simulink model "sliding_mode_controller_2014b"  (R2021b)
settings: Solver=ode3  StartTime=0.0  StopTime=30  FixedStep=0.01  RelTol=1e-3  EnableMultiTasking=on
model workspace (MAT data in the model file):
  P_C_1 = Simulink.Signal
  P_C_1.DataType = 'double'
  P_C_1.Dimensions = 1
  P_C_1.DimensionsMode = 'Fixed'
  P_C_1.Complexity = 'real'
  P_C_1.SampleTime = -1
  P_C_1.SamplingMode = 'Sample based'
  P_C_1.InitialValue = '0'
  P_C_2 = Simulink.Signal
  P_C_2.DataType = 'double'
  P_C_2.Dimensions = 1
  P_C_2.DimensionsMode = 'Fixed'
  P_C_2.Complexity = 'real'
  P_C_2.SampleTime = -1
  P_C_2.SamplingMode = 'Sample based'
  P_C_2.InitialValue = '0'
  P_C_3 = Simulink.Signal
  P_C_3.DataType = 'double'
  P_C_3.Dimensions = 1
  P_C_3.DimensionsMode = 'Fixed'
  P_C_3.Complexity = 'real'
  P_C_3.SampleTime = -1
  P_C_3.SamplingMode = 'Sample based'
  P_C_3.InitialValue = '0'
  P_C_4 = Simulink.Signal
  P_C_4.DataType = 'double'
  P_C_4.Dimensions = 1
  P_C_4.DimensionsMode = 'Fixed'
  P_C_4.Complexity = 'real'
  P_C_4.SampleTime = -1
  P_C_4.SamplingMode = 'Sample based'
  P_C_4.InitialValue = '0'
  alfa_1 = Simulink.Signal
  alfa_1.DataType = 'double'
  alfa_1.Dimensions = 1
  alfa_1.DimensionsMode = 'Fixed'
  alfa_1.Complexity = 'real'
  alfa_1.SampleTime = -1
  alfa_1.SamplingMode = 'Sample based'
  alfa_1.InitialValue = '0'
  alfa_2 = Simulink.Signal
  alfa_2.DataType = 'double'
  alfa_2.Dimensions = 1
  alfa_2.DimensionsMode = 'Fixed'
  alfa_2.Complexity = 'real'
  alfa_2.SampleTime = -1
  alfa_2.SamplingMode = 'Sample based'
  alfa_2.InitialValue = '0'
  alfa_3 = Simulink.Signal
  alfa_3.DataType = 'double'
  alfa_3.Dimensions = 1
  alfa_3.DimensionsMode = 'Fixed'
  alfa_3.Complexity = 'real'
  alfa_3.SampleTime = -1
  alfa_3.SamplingMode = 'Sample based'
  alfa_3.InitialValue = '0'
  counter_1 = Simulink.Signal
  counter_1.DataType = 'double'
  counter_1.Dimensions = 1
  counter_1.DimensionsMode = 'Fixed'
  counter_1.Complexity = 'real'
  counter_1.SampleTime = -1
  counter_1.SamplingMode = 'Sample based'
  counter_1.InitialValue = '0'
  counter_2 = Simulink.Signal
  counter_2.DataType = 'double'
  counter_2.Dimensions = 1
  counter_2.DimensionsMode = 'Fixed'
  counter_2.Complexity = 'real'
  counter_2.SampleTime = -1
  counter_2.SamplingMode = 'Sample based'
  counter_2.InitialValue = '0'
  counter_3 = Simulink.Signal
  counter_3.DataType = 'double'
  counter_3.Dimensions = 1
  counter_3.DimensionsMode = 'Fixed'
  counter_3.Complexity = 'real'
  counter_3.SampleTime = -1
  counter_3.SamplingMode = 'Sample based'
  counter_3.InitialValue = '0'
  counter_4 = Simulink.Signal
  counter_4.DataType = 'double'
  counter_4.Dimensions = 1
  counter_4.DimensionsMode = 'Fixed'
  counter_4.Complexity = 'real'
  counter_4.SampleTime = -1
  counter_4.SamplingMode = 'Sample based'
  counter_4.InitialValue = '0'
  lambda_1 = Simulink.Signal
  lambda_1.DataType = 'double'
  lambda_1.Dimensions = 1
  lambda_1.DimensionsMode = 'Fixed'
  lambda_1.Complexity = 'real'
  lambda_1.SampleTime = -1
  lambda_1.SamplingMode = 'Sample based'
  lambda_1.InitialValue = '0'
  lambda_2 = Simulink.Signal
  lambda_2.DataType = 'double'
  lambda_2.Dimensions = 1
  lambda_2.DimensionsMode = 'Fixed'
  lambda_2.Complexity = 'real'
  lambda_2.SampleTime = -1
  lambda_2.SamplingMode = 'Sample based'
  lambda_2.InitialValue = '0'
  lambda_3 = Simulink.Signal
  lambda_3.DataType = 'double'
  lambda_3.Dimensions = 1
  lambda_3.DimensionsMode = 'Fixed'
  lambda_3.Complexity = 'real'
  lambda_3.SampleTime = -1
  lambda_3.SamplingMode = 'Sample based'
  lambda_3.InitialValue = '0'
  mf_1 = Simulink.Signal
  mf_1.DataType = 'double'
  mf_1.Dimensions = 1
  mf_1.DimensionsMode = 'Fixed'
  mf_1.Complexity = 'real'
  mf_1.SampleTime = -1
  mf_1.SamplingMode = 'Sample based'
  mf_1.InitialValue = '.5'
  mf_2 = Simulink.Signal
  mf_2.DataType = 'double'
  mf_2.Dimensions = 1
  mf_2.DimensionsMode = 'Fixed'
  mf_2.Complexity = 'real'
  mf_2.SampleTime = -1
  mf_2.SamplingMode = 'Sample based'
  mf_2.InitialValue = '.5'
  mf_3 = Simulink.Signal
  mf_3.DataType = 'double'
  mf_3.Dimensions = 1
  mf_3.DimensionsMode = 'Fixed'
  mf_3.Complexity = 'real'
  mf_3.SampleTime = -1
  mf_3.SamplingMode = 'Sample based'
  mf_3.InitialValue = '.5'
  step_counter = Simulink.Signal
  step_counter.DataType = 'double'
  step_counter.Dimensions = 1
  step_counter.DimensionsMode = 'auto'
  step_counter.Complexity = 'real'
  step_counter.SampleTime = -1
  step_counter.SamplingMode = 'auto'
  step_counter.InitialValue = '0'
  trans_b_1 = Simulink.Signal
  trans_b_1.DataType = 'double'
  trans_b_1.Dimensions = 1
  trans_b_1.DimensionsMode = 'Fixed'
  trans_b_1.Complexity = 'real'
  trans_b_1.SampleTime = -1
  trans_b_1.SamplingMode = 'Sample based'
  trans_b_1.InitialValue = '0'
  trans_b_2 = Simulink.Signal
  trans_b_2.DataType = 'double'
  trans_b_2.Dimensions = 1
  trans_b_2.DimensionsMode = 'Fixed'
  trans_b_2.Complexity = 'real'
  trans_b_2.SampleTime = -1
  trans_b_2.SamplingMode = 'Sample based'
  trans_b_2.InitialValue = '0'
  trans_b_3 = Simulink.Signal
  trans_b_3.DataType = 'double'
  trans_b_3.Dimensions = 1
  trans_b_3.DimensionsMode = 'Fixed'
  trans_b_3.Complexity = 'real'
  trans_b_3.SampleTime = -1
  trans_b_3.SamplingMode = 'Sample based'
  trans_b_3.InitialValue = '0'
  trans_b_4 = Simulink.Signal
  trans_b_4.DataType = 'double'
  trans_b_4.Dimensions = 1
  trans_b_4.DimensionsMode = 'Fixed'
  trans_b_4.Complexity = 'real'
  trans_b_4.SampleTime = -1
  trans_b_4.SamplingMode = 'Sample based'
  trans_b_4.InitialValue = '0'
values from neighbouring files (symbols this model uses):
  alfa0 = 15*pi/180    (= 0.261799387799)    [engine_initials_smc.m]
  etaif2 = -0.015    [engine_initials_smc.m]
  Hu = 43000    [engine_initials_smc.m]
  I = Iac*(2.0*pi/60)^2*1000    (= 5.26378901391)    [engine_initials_smc.m]
  kb2 = 0.470    (= 0.47)    [engine_initials_smc.m]
  Lth = 14.67    [engine_initials_smc.m]
  mat1 = 5.9403    [engine_initials_smc.m]
  Ncyl = 4    [engine_initials_smc.m]
  Pa = 1.013    [engine_initials_smc.m]
  Pc = .4125    (= 0.4125)    [engine_initials_smc.m]
  R = 0.00287    [engine_initials_smc.m]
  si = .961    (= 0.961)    [engine_initials_smc.m]
  Ta = 293    [engine_initials_smc.m]
  Ti = 308    [engine_initials_smc.m]
  Vd = 1.275    [engine_initials_smc.m]
  Vi = 3*564e-6    (= 0.001692)    [engine_initials_smc.m]
  yi = -0.07    [engine_initials_smc.m]
undefined symbols (not defined in the file or in its folder): sigbuilder_block
settings Model: Creator=Tohid SA  LastModifiedBy=12143
settings SolverCC: ZeroCrossAlgorithm=Adaptive  AlgebraicLoopSolver=TrustRegion
settings DataIOCC: SaveFormat=Array  SignalLoggingSaveFormat=ModelDataLogs  SaveOutput=off  ReturnWorkspaceOutputs=off
settings OptimizationCC: ExpressionDepthLimit=2147483647  LifeSpan=inf
settings DebuggingCC: UnderspecifiedInitializationDetection=Classic  MergeDetectMultiDrivingBlocksExec=none  SolverPrmCheckMsg=warning  FcnCallInpInsideContextMsg=warning  StateNameClashWarn=warning  SFUnexpectedBacktrackingDiag=warning  SFNoUnconditionalDefaultTransitionDiag=warning  SFExecutionAtInitializationDiag=none  SFMachineParentedDataDiag=warning  ArithmeticOperatorsInVariantConditions=warning
settings HardwareCC: ProdBitPerPointer=32  ProdBitPerSizeT=32  ProdBitPerPtrDiffT=32  ProdLargestAtomicFloat=None  ProdIntDivRoundTo=Undefined  ProdEndianess=Unspecified  ProdWordSize=32  ProdHWDeviceType=32-bit Generic
settings ModelReferenceCC: PropagateSignalLabelsOutOfModel=off
settings SFSimCC: SimUseLocalCustomCode=off  CustomCodeUndefinedFunction=UseInterfaceOnly
settings RTWCC: RTWUseLocalCustomCode=off
settings CodeAppCC: StateflowObjectComments=on
settings GRTTargetCC: TargetLangStandard=C89/C90 (ANSI)  CombineOutputUpdateFcns=off  GRTInterface=on
settings ConfigComp: CovMetricSettings=dw  CovSaveCumulativeToWorkspaceVar=on  CovSaveSingleToWorkspaceVar=on  CovExternalEMLEnable=off

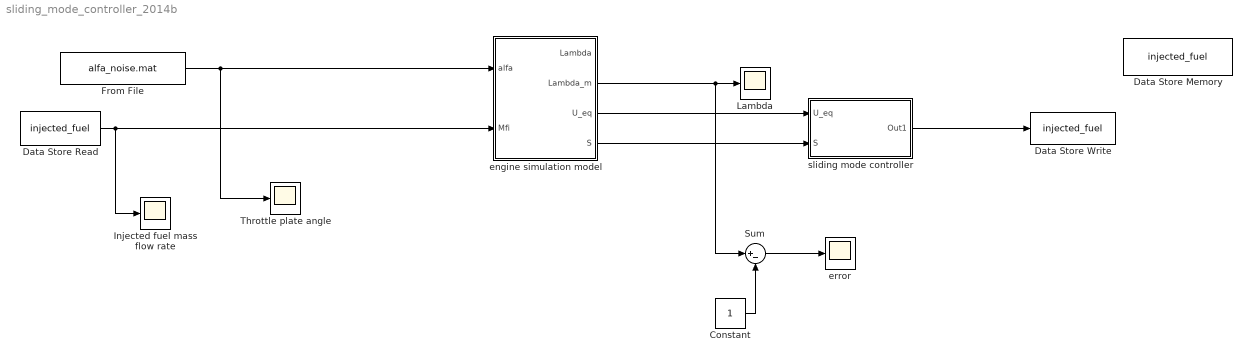
== system sliding_mode_controller_2014b ==
  Constant : Constant
  Data Store Memory : DataStoreMemory  DataStoreName=injected_fuel  ReadBeforeWriteMsg=warning  WriteAfterWriteMsg=warning  WriteAfterReadMsg=warning  InitialValue=0.0079  ShowAdditionalParam=off
  Data Store Read : DataStoreRead  DataStoreName=injected_fuel  IndexOptions=Index vector (dialog)  Indices=1  OutputSizes=1
  Data Store Write : DataStoreWrite  DataStoreName=injected_fuel  IndexOptions=Index vector (dialog)  Indices=1  OutputSizes=1
  From File : FromFile  FileName=alfa_noise.mat
  Injected fuel mass flow rate : Scope
  Lambda : Scope
  Sum : Sum  Inputs=|+-
  Throttle plate angle : Scope
  engine simulation model : Subsystem
  error : Scope
  sliding mode controller : Subsystem
  wires:
  engine simulation model/3(U_eq) -> sliding mode controller/1(U_eq)
  engine simulation model/4(S) -> sliding mode controller/2(S)
  sliding mode controller/1(Out1) -> Data Store Write/1
  Data Store Read/1 -> Injected fuel mass flow rate/1, engine simulation model/2(Mfi)
  From File/1 -> engine simulation model/1(alfa), Throttle plate angle/1
  engine simulation model/2(Lambda_m) -> Lambda/1, Sum/1
  Constant/1 -> Sum/2
  Sum/1 -> error/1

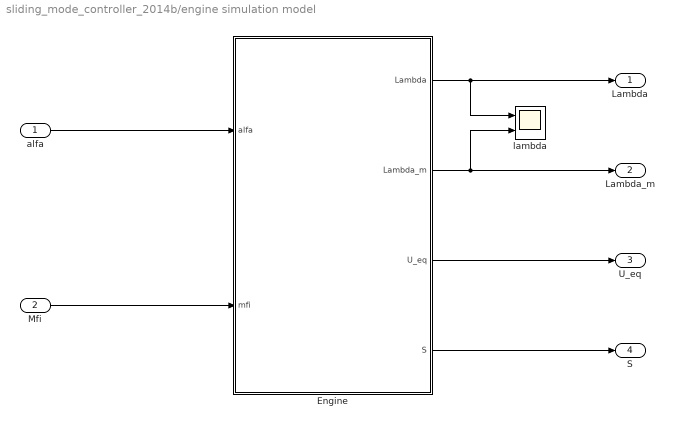
== system sliding_mode_controller_2014b/engine simulation model ==
  alfa : Inport
  Mfi : Inport  Port=2
  Engine : Subsystem
  lambda : Scope  NumInputPorts=2
  Lambda : Outport
  Lambda_m : Outport  Port=2
  U_eq : Outport  Port=3
  S : Outport  Port=4
  wires:
  Engine/1(Lambda) -> lambda/1, Lambda/1
  alfa/1 -> Engine/1(alfa)
  Mfi/1 -> Engine/2(mfi)
  Engine/2(Lambda_m) -> lambda/2, Lambda_m/1
  Engine/3(U_eq) -> U_eq/1
  Engine/4(S) -> S/1

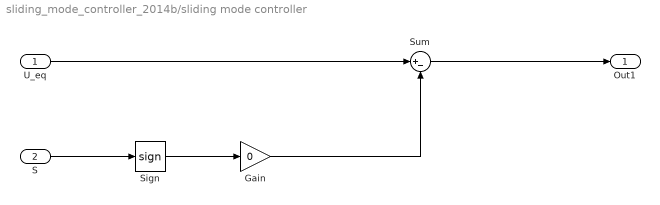
== system sliding_mode_controller_2014b/sliding mode controller ==
  U_eq : Inport
  S : Inport  Port=2
  Gain : Gain  Gain=0
  Sign : Signum
  Sum : Sum  Inputs=|+-
  Out1 : Outport
  wires:
  U_eq/1 -> Sum/1
  S/1 -> Sign/1
  Sign/1 -> Gain/1
  Gain/1 -> Sum/2
  Sum/1 -> Out1/1

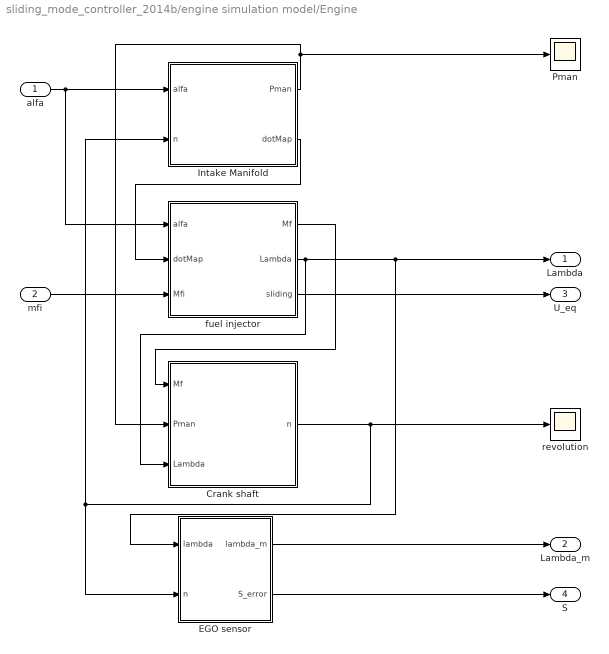
== system sliding_mode_controller_2014b/engine simulation model/Engine ==
  alfa : Inport
  mfi : Inport  Port=2
  "Crank shaft " : Subsystem
  EGO sensor : Subsystem
  Intake Manifold : Subsystem
  Pman : Scope
  fuel injector : Subsystem
  revolution : Scope
  Lambda : Outport
  Lambda_m : Outport  Port=2
  U_eq : Outport  Port=3
  S : Outport  Port=4
  wires:
  alfa/1 -> Intake Manifold/1(alfa), fuel injector/1(alfa)
  "Crank shaft "/1(n) -> revolution/1, Intake Manifold/2(n), EGO sensor/2(n)
  Intake Manifold/1(Pman) -> Pman/1, "Crank shaft "/2(Pman)
  Intake Manifold/2(dotMap) -> fuel injector/2(dotMap)
  fuel injector/1(Mf) -> "Crank shaft "/1(Mf)
  fuel injector/2(Lambda) -> "Crank shaft "/3(Lambda), Lambda/1, EGO sensor/1(lambda)
  mfi/1 -> fuel injector/3(Mfi)
  EGO sensor/1(lambda_m) -> Lambda_m/1
  fuel injector/3("sliding ") -> U_eq/1
  EGO sensor/2(S_error) -> S/1

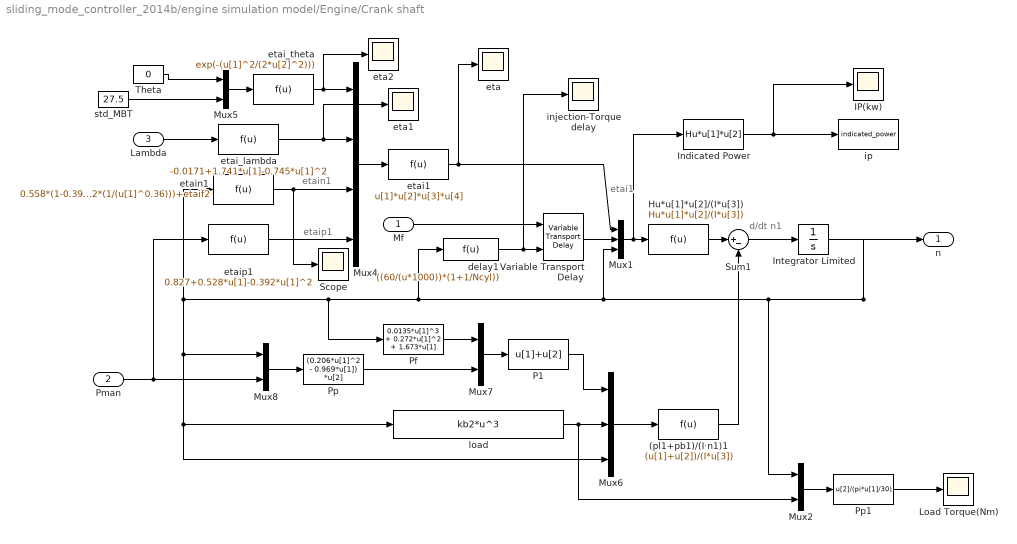
== system sliding_mode_controller_2014b/engine simulation model/Engine/Crank shaft  ==
  note: d/dt n1
  note: etai1
  note: etain1
  note: etaip1
  Mf : Inport
  Pman : Inport  Port=2
  Lambda : Inport  Port=3
  (pl1+pb1)/(I·n1)1 : Fcn  Expr=(u[1]+u[2])/(I*u[3])
  Hu*u[1]*u[2]/(I*u[3]) : Fcn  Expr=Hu*u[1]*u[2]/(I*u[3])
  IP(kw) : Scope
  Indicated Power : Fcn  Expr=Hu*u[1]*u[2]
  Integrator Limited : Integrator  InitialCondition=3.75  LimitOutput=on
  Load Torque(Nm) : Scope
  Mux1 : Mux  Inputs=3
  Mux{2,5,7..8} (4 alike) : Mux  Inputs=2
  Mux4 : Mux
  Mux6 : Mux  Inputs=3
  P1 : Fcn  Expr=u[1]+u[2]
  Pf : Fcn  Expr=0.0135*u[1]^3 + 0.272*u[1]^2 + 1.673*u[1]
  Pp : Fcn  Expr=(0.206*u[1]^2 - 0.969*u[1]) *u[2]
  Pp1 : Fcn  Expr=u[2]/(pi*u[1]/30)
  Scope : Scope
  Sum1 : Sum  Inputs=|+-  InputSameDT=on  SaturateOnIntegerOverflow=on  OutDataTypeStr=Inherit: Same as first input
  Theta : Constant  Value=0
  Variable Transport Delay : VariableTransportDelay  MaximumDelay=10  MaximumPoints=40000  ZeroDelay=on
  delay1 : Fcn  Expr=((60/(u*1000))*(1+1/Ncyl))
  eta : Scope
  eta1 : Scope
  eta2 : Scope
  etai1 : Fcn  Expr=u[1]*u[2]*u[3]*u[4]
  etai_lambda : Fcn  Expr=-0.0171+1.741*u[1]-0.745*u[1]^2
  etai_theta : Fcn  Expr=exp(-(u[1]^2/(2*u[2]^2)))
  etain1 : Fcn  Expr=0.558*(1-0.392*(1/(u[1]^0.36)))+etaif2
  etaip1 : Fcn  Expr=0.827+0.528*u[1]-0.392*u[1]^2
  injection-Torque delay : Scope
  ip : ToWorkspace  VariableName=indicated_power  SampleTime=-1
  load : Fcn  Expr=kb2*u^3
  std_MBT : Constant  Value=27.5
  n : Outport
  wires:
  Hu*u[1]*u[2]/(I*u[3])/1 -> Sum1/1
  Mux1/1 -> Hu*u[1]*u[2]/(I*u[3])/1, Indicated Power/1
  Sum1/1 -> Integrator Limited/1
  Integrator Limited/1 -> n/1, Mux1/3, Pf/1, etain1/1, Mux8/1, Mux6/3, load/1, delay1/1, Mux2/1
  Mux4/1 -> etai1/1
  etai_theta/1 -> Mux4/1, eta2/1
  etai_lambda/1 -> Mux4/2, eta1/1
  std_MBT/1 -> Mux5/2
  Theta/1 -> Mux5/1
  Mux5/1 -> etai_theta/1
  Lambda/1 -> etai_lambda/1
  etai1/1 -> Mux1/1, eta/1
  etain1/1 -> Mux4/3, Scope/1
  etaip1/1 -> Mux4/4
  Pman/1 -> etaip1/1, Mux8/2
  P1/1 -> Mux6/1
  Mux7/1 -> P1/1
  Pf/1 -> Mux7/1
  Pp/1 -> Mux7/2
  Mux8/1 -> Pp/1
  load/1 -> Mux6/2, Mux2/2
  Mux6/1 -> (pl1+pb1)/(I·n1)1/1
  (pl1+pb1)/(I·n1)1/1 -> Sum1/2
  Variable Transport Delay/1 -> Mux1/2
  delay1/1 -> injection-Torque delay/1, Variable Transport Delay/2
  Indicated Power/1 -> ip/1, IP(kw)/1
  Mux2/1 -> Pp1/1
  Pp1/1 -> Load Torque(Nm)/1
  Mf/1 -> Variable Transport Delay/1

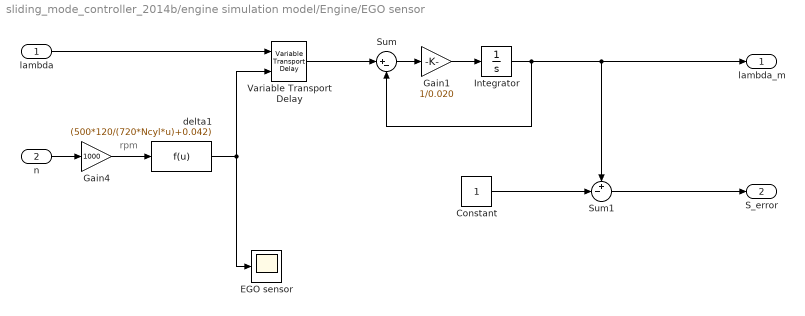
== system sliding_mode_controller_2014b/engine simulation model/Engine/EGO sensor ==
  note: rpm
  lambda : Inport
  n : Inport  Port=2
  Constant : Constant
  EGO sensor : Scope
  Gain1 : Gain  Gain=1/0.020
  Gain4 : Gain  Gain=1000
  Integrator : Integrator  InitialCondition=1.02
  Sum : Sum  Inputs=|+-
  Sum1 : Sum  Inputs=+-|
  Variable Transport Delay : VariableTransportDelay  MaximumDelay=10  MaximumPoints=40000
  delta1 : Fcn  Expr=(500*120/(720*Ncyl*u)+0.042)
  lambda_m : Outport
  S_error : Outport  Port=2
  wires:
  Sum/1 -> Gain1/1
  Gain1/1 -> Integrator/1
  Integrator/1 -> Sum/2, lambda_m/1, Sum1/1
  n/1 -> Gain4/1
  Gain4/1 -> delta1/1
  delta1/1 -> EGO sensor/1, Variable Transport Delay/2
  lambda/1 -> Variable Transport Delay/1
  Variable Transport Delay/1 -> Sum/1
  Constant/1 -> Sum1/2
  Sum1/1 -> S_error/1

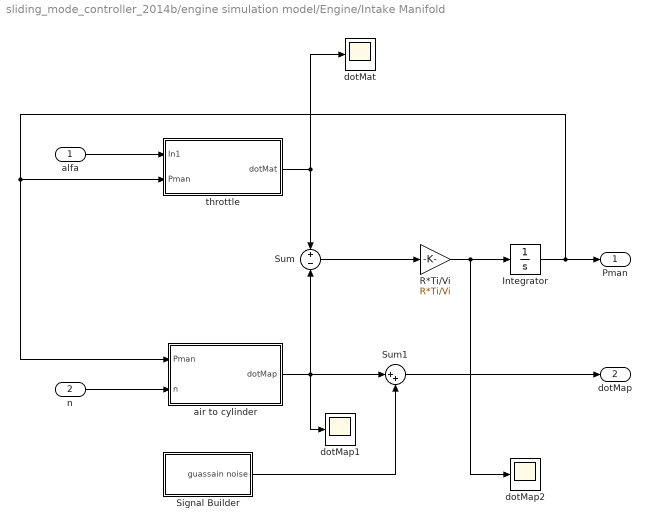
== system sliding_mode_controller_2014b/engine simulation model/Engine/Intake Manifold ==
  alfa : Inport
  n : Inport  Port=2
  Integrator : Integrator  InitialCondition=1.733
  R*Ti/Vi : Gain  Gain=R*Ti/Vi
  Signal Builder : Subsystem  Tag=STV Subsys  LoadFcn=sigbuilder_block('load');  StartFcn=sigbuilder_block('start');  StopFcn=sigbuilder_block('stop');  ClipboardFcn=sigbuilder_block('clipboard');  mask(Sigbuilder block){tuvar=[0:10]}
      mask help: Create and generate interchangeable groups of signals whose waveforms are piecewise linear.
      mask init:
      | if ~strcmp(get_param(bdroot(gcbh),'SimulationStatus'),'stopped') tuvar = sigbuilder_block('maskInit'); end
      settings: CopyFcn=sigbuilder_block('copy');  DeleteFcn=sigbuilder_block('delete');  ModelCloseFcn=sigbuilder_block('modelClose');  PreSaveFcn=sigbuilder_block('preSave');  PauseFcn=sigbuilder_block('pause')  ContinueFcn=sigbuilder_block('continue')  NameChangeFcn=sigbuilder_block('namechange');  OpenFcn=sigbuilder_block('open',[0 30 1024.5 489 ]);  CloseFcn=sigbuilder_block('close');
      mask Display: plot(0, 0, 100, 100,[2, 2, 32, 32, 2], [68, 8, 8, 68, 68],[32, 2], [38, 38], [32, 19, 2],[53, 60, 44], [32, 17, 17, 2],[16, 16, 31, 31]);txt = getActiveGroup(gcbh);text(2, 100, txt,'verticalAlignment', 'top');
  Sum : Sum  Inputs=+|-
  Sum1 : Sum  Inputs=|++
  air to cylinder : Subsystem
  dotMap1 : Scope
  dotMap2 : Scope
  dotMat : Scope
  throttle : Subsystem
  Pman : Outport
  dotMap : Outport  Port=2
  wires:
  alfa/1 -> throttle/1(In1)
  air to cylinder/1(dotMap) -> Sum/2, dotMap1/1, Sum1/1
  throttle/1(dotMat) -> Sum/1, dotMat/1
  Sum/1 -> R*Ti/Vi/1
  R*Ti/Vi/1 -> Integrator/1, dotMap2/1
  Integrator/1 -> Pman/1, throttle/2(Pman), air to cylinder/1(Pman)
  n/1 -> air to cylinder/2(n)
  Signal Builder/1("guassain noise ") -> Sum1/2
  Sum1/1 -> dotMap/1

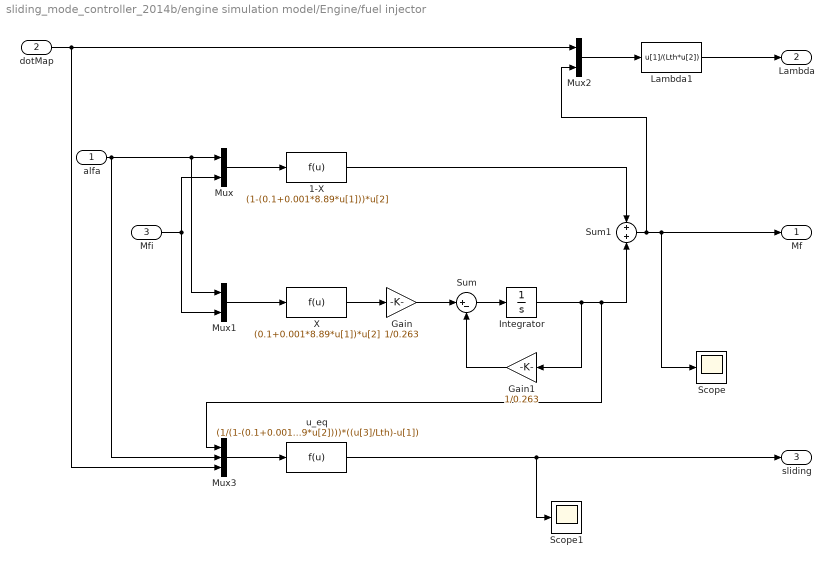
== system sliding_mode_controller_2014b/engine simulation model/Engine/fuel injector ==
  alfa : Inport
  dotMap : Inport  Port=2
  Mfi : Inport  Port=3
  1-X : Fcn  Expr=(1-(0.1+0.001*8.89*u[1]))*u[2]
  Gain : Gain  Gain=1/0.263
  Gain1 : Gain  Gain=1/0.263
  Integrator : Integrator  InitialCondition=0.1  UpperSaturationLimit=0.0079  LowerSaturationLimit=.0001
  Lambda1 : Fcn  Expr=u[1]/(Lth*u[2])
  Mux : Mux  Inputs=2
  Mux1 : Mux  Inputs=2
  Mux2 : Mux  Inputs=2
  Mux3 : Mux  Inputs=3
  Scope : Scope
  Scope1 : Scope
  Sum : Sum  Inputs=|+-
  Sum1 : Sum  Inputs=+|+
  X : Fcn  Expr=(0.1+0.001*8.89*u[1])*u[2]
  u_eq : Fcn  Expr=(1/(1-(0.1+0.001*8.89*u[2])))*((u[3]/Lth)-u[1])
  Mf : Outport
  Lambda : Outport  Port=2
  "sliding " : Outport  Port=3
  wires:
  alfa/1 -> Mux1/1, Mux/1, Mux3/2
  Mfi/1 -> Mux1/2, Mux/2
  Mux1/1 -> X/1
  X/1 -> Gain/1
  Gain/1 -> Sum/1
  Sum/1 -> Integrator/1
  Integrator/1 -> Gain1/1, Sum1/2, Mux3/1
  Gain1/1 -> Sum/2
  Mux/1 -> 1-X/1
  1-X/1 -> Sum1/1
  Sum1/1 -> Mux2/2, Mf/1, Scope/1
  dotMap/1 -> Mux2/1, Mux3/3
  Mux2/1 -> Lambda1/1
  Lambda1/1 -> Lambda/1
  Mux3/1 -> u_eq/1
  u_eq/1 -> Scope1/1, "sliding "/1

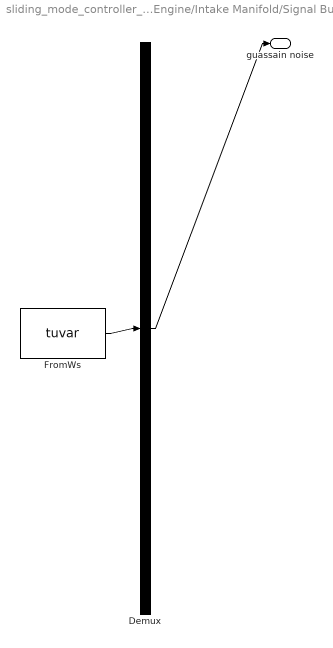
== system sliding_mode_controller_2014b/engine simulation model/Engine/Intake Manifold/Signal Builder ==
  Demux : Demux  Tag=STV Demux  Outputs=1
      settings: DisplayOption=none
  FromWs : FromWorkspace  Tag=STV FromWs  VariableName=tuvar
      SigBuilderData=|
      | common.afterFinalStr = 'Extrapolate'
      | common.sampleTime = 0
      | dataSet.timeRange = [0 30]
      | dataSet.name = 'Group 1'
      | sbobj.Groups.Name = 'Group 1'
      | sbobj.Groups.Signals.Name = 'guassain noise '
      | sbobj.Groups.Signals.XData = [0 0.1 0.2 0.3 0.4 0.5 0.6 0.7 0.8 0.9 1 1.1 1.2 1.3 1.4 1.5 1.6 1.7 1.8 1.9 2 2.1 2.2 2.3 2.4 2.5 2.6 2.7 2.8 2.9 3 3.1 3.2 3.3 3.4 3.5 3.6 3.7 3.8 3.9 4 4.1 4.2 4.3 4.4 4.5 4.6 4.7 4.8 4.9 5 5.1 5.2 5.3 5.4 5.5 5.6 5.7 5.8 5.9 6 6.1 6.2 6.3 6.4 6.5 6.6 6.7 6.8 6.9 7 7.1 7.2 7.3 7.4 7.5 7.6 7.7 7.8 7.9 8 8.1 8.2 8.3 8.4 8.5 8.6 8.7 8.8 8.9 9 9.1 9.2 9.3 9.4 9.5 9.6 9.7 9.8 9.9 10 10.1 10.2 10.3 10.4 10.5 10.6 10.7 10.8 10.9 11 11.1 11.2 11.3 11.4 11.5 11.6 11.7 11.8 11.9 12 12.1 12.2 12.3 12.4 12.5 12.6 12.7 12.8 12.9 13 13.1 13.2 13.3 13.4 13.5 13.6 13.7 13.8 13.9 14 14.1 14.2 14.3 14.4 14.5 14.6 14.7 14.8 14.9 15 15.1 15.2 15.3 15.4 15.5 15.6 15.7 15.8 15.9 16 16.1 16.2 16.3 16.4 16.5 16.6 16.7 16.8 16.9 17 17.1 17.2 17.3 17.4 17.5 17.6 17.7 17.8 17.9 18 18.1 18.2 18.3 18.4 18.5 18.6 18.7 18.8 18.9 19 19.1 19.2 19.3 19.4 19.5 19.6 19.7 19.8 19.9 20 20.1 20.2 20.3 20.4 20.5 20.6 20.7 20.8 20.9 21 21.1 21.2 21.3 21.4 21.5 21.6 21.7 21.8 21.9 22 22.1 22.2 22.3 22.4 22.5 22.6 22.7 22.8 22.9 23 23.1 23.2 23.3 23.4 23.5 23.6 23.7 23.8 23.9 24 24.1 24.2 24.3 24.4 24.5 24.6 24.7 24.8 24.9 25 25.1 25.2 25.3 25.4 25.5 25.6 25.7 25.8 25.9 26 26.1 26.2 26.3 26.4 26.5 26.6 26.7 26.8 26.9 27 27.1 27.2 27.3 27.4 27.5 27.6 27.7 27.8 27.9 28 28.1 28.2 28.3 28.4 28.5 28.6 28.7 28.8 28.9 29 29.1 29.2 29.3 29.4 29.5 29.6 29.7 29.8 29.9 30]
      | sbobj.Groups.Signals.YData = [-0.00505489732513 -0.00245532881445 0.00153127824542 -0.000137215324972 -0.00279683000613 -0.00156594634717 0.000623794351407 -0.00248254751637 0.00243737556203 -0.00160177376682 0.0045221565513 -0.00269966562685 ... (301 elements, 1x301)]
      | sbobj.Groups.TimeRange = [0 30]
  "guassain noise " : Outport  Tag=STV Outport
  wires:
  FromWs/1 -> Demux/1
  Demux/1 -> "guassain noise "/1

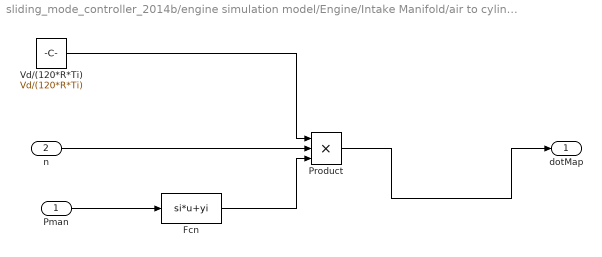
== system sliding_mode_controller_2014b/engine simulation model/Engine/Intake Manifold/air to cylinder ==
  Pman : Inport
  n : Inport  Port=2
  Fcn : Fcn  Expr=si*u+yi
  Product : Product  Inputs=3  RndMeth=Zero
  Vd/(120*R*Ti) : Constant  Value=Vd/(120*R*Ti)
  dotMap : Outport
  wires:
  Pman/1 -> Fcn/1
  Fcn/1 -> Product/3
  n/1 -> Product/2
  Vd/(120*R*Ti)/1 -> Product/1
  Product/1 -> dotMap/1

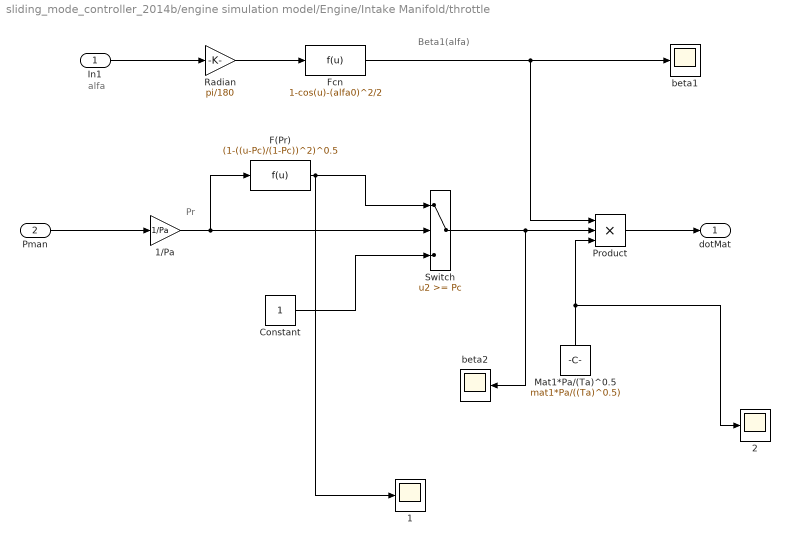
== system sliding_mode_controller_2014b/engine simulation model/Engine/Intake Manifold/throttle ==
  note: Beta1(alfa)
  note: alfa
  note: Pr
  In1 : Inport
  Pman : Inport  Port=2
  1 : Scope
  1/Pa : Gain  Gain=1/Pa
  2 : Scope
  Constant : Constant
  F(Pr) : Fcn  Expr=(1-((u-Pc)/(1-Pc))^2)^0.5
  Fcn : Fcn  Expr=1-cos(u)-(alfa0)^2/2
  Mat1*Pa/(Ta)^0.5 : Constant  Value=mat1*Pa/((Ta)^0.5)
  Product : Product  Inputs=3  RndMeth=Zero
  Radian : Gain  Gain=pi/180
  Switch : Switch  Threshold=Pc
  beta1 : Scope
  beta2 : Scope
  dotMat : Outport
  wires:
  In1/1 -> Radian/1
  Radian/1 -> Fcn/1
  Fcn/1 -> beta1/1, Product/1
  Mat1*Pa/(Ta)^0.5/1 -> Product/3, 2/1
  Product/1 -> dotMat/1
  Pman/1 -> 1/Pa/1
  1/Pa/1 -> F(Pr)/1, Switch/2
  F(Pr)/1 -> Switch/1, 1/1
  Constant/1 -> Switch/3
  Switch/1 -> Product/2, beta2/1
